simulink model "EL6243_Project_Simulink"  (R2013a)
settings: Solver=ode45  StartTime=0.0  StopTime=60  RelTol=1e-3
libraries: cstblocks x12
settings Model: Creator=pk  LastModifiedBy=meetm_000
settings DataIOCC: SignalLoggingSaveFormat=ModelDataLogs
settings OptimizationCC: InitFltsAndDblsToZero=on
settings DebuggingCC: SaveWithParameterizedLinksMsg=none  SignalResolutionControl=TryResolveAllWithWarning  MultiTaskDSMMsg=warning  MultiTaskCondExecSysMsg=none  StrictBusMsg=None
settings RTWCC: IncludeERTFirstTime=on
settings GRTTargetCC: TargetFcnLib=ansi_tfl_tmw.mat  CombineOutputUpdateFcns=off  GRTInterface=on

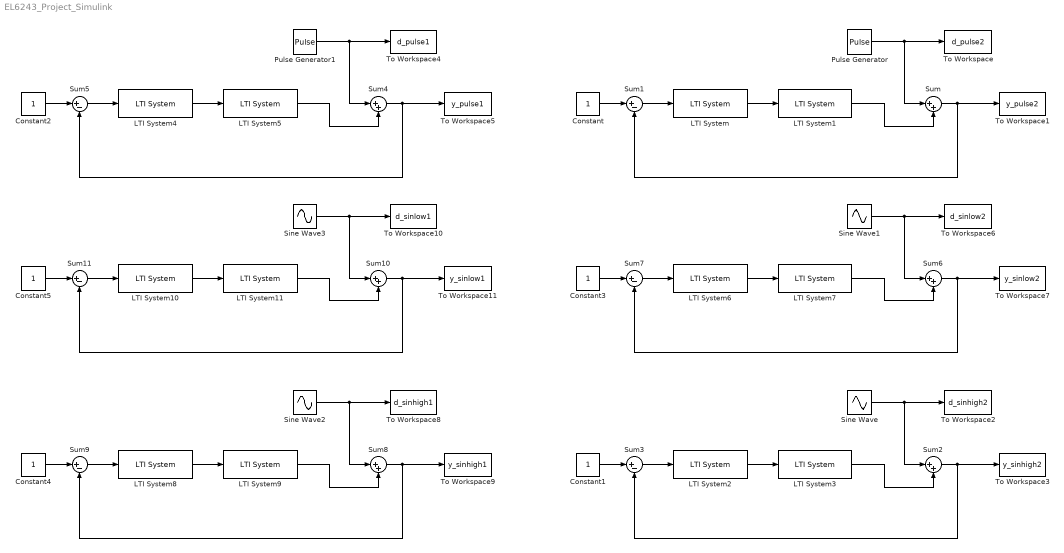
== system EL6243_Project_Simulink ==
  Constant{,1..5} (6 alike) : Constant
  LTI System : cstblocks/LTI System  sys=Gco  IC=[]
  LTI System{1,3,5,7,9,11} (6 alike) : cstblocks/LTI System  sys=Gp  IC=[]
  LTI System10 : cstblocks/LTI System  sys=Gc  IC=[]
  LTI System2 : cstblocks/LTI System  sys=Gco  IC=[]
  LTI System4 : cstblocks/LTI System  sys=Gc  IC=[]
  LTI System6 : cstblocks/LTI System  sys=Gco  IC=[]
  LTI System8 : cstblocks/LTI System  sys=Gc  IC=[]
  Pulse Generator : DiscretePulseGenerator  PulseType=Time based  Period=100  PhaseDelay=40
  Pulse Generator1 : DiscretePulseGenerator  PulseType=Time based  Period=100  PhaseDelay=40
  Sine Wave : Sin  Frequency=10*pi  SampleTime=0
  Sine Wave1 : Sin  Amplitude=0.2  SampleTime=0
  Sine Wave2 : Sin  Frequency=10*pi  SampleTime=0
  Sine Wave3 : Sin  Amplitude=0.2  SampleTime=0
  Sum{,2,4,6,8,10} (6 alike) : Sum  Inputs=|++
  Sum{1,3,5,7,9,11} (6 alike) : Sum  Inputs=|+-
  To Workspace : ToWorkspace  VariableName=d_pulse2  SampleTime=0.01  SaveFormat=Structure With Time
  To Workspace1 : ToWorkspace  VariableName=y_pulse2  SampleTime=0.01  SaveFormat=Structure With Time
  To Workspace10 : ToWorkspace  VariableName=d_sinlow1  SampleTime=0.01  SaveFormat=Structure With Time
  To Workspace11 : ToWorkspace  VariableName=y_sinlow1  SampleTime=0.01  SaveFormat=Structure With Time
  To Workspace2 : ToWorkspace  VariableName=d_sinhigh2  SampleTime=0.01  SaveFormat=Structure With Time
  To Workspace3 : ToWorkspace  VariableName=y_sinhigh2  SampleTime=0.01  SaveFormat=Structure With Time
  To Workspace4 : ToWorkspace  VariableName=d_pulse1  SampleTime=0.01  SaveFormat=Structure With Time
  To Workspace5 : ToWorkspace  VariableName=y_pulse1  SampleTime=0.01  SaveFormat=Structure With Time
  To Workspace6 : ToWorkspace  VariableName=d_sinlow2  SampleTime=0.01  SaveFormat=Structure With Time
  To Workspace7 : ToWorkspace  VariableName=y_sinlow2  SampleTime=0.01  SaveFormat=Structure With Time
  To Workspace8 : ToWorkspace  VariableName=d_sinhigh1  SampleTime=0.01  SaveFormat=Structure With Time
  To Workspace9 : ToWorkspace  VariableName=y_sinhigh1  SampleTime=0.01  SaveFormat=Structure With Time
  wires:
  LTI System/1 -> LTI System1/1
  LTI System1/1 -> Sum/2
  Pulse Generator/1 -> To Workspace/1, Sum/1
  Constant/1 -> Sum1/1
  Sum1/1 -> LTI System/1
  Sum/1 -> To Workspace1/1, Sum1/2
  LTI System2/1 -> LTI System3/1
  LTI System3/1 -> Sum2/2
  Sine Wave/1 -> To Workspace2/1, Sum2/1
  Constant1/1 -> Sum3/1
  Sum3/1 -> LTI System2/1
  Sum2/1 -> To Workspace3/1, Sum3/2
  LTI System6/1 -> LTI System7/1
  LTI System7/1 -> Sum6/2
  Sine Wave1/1 -> To Workspace6/1, Sum6/1
  Constant3/1 -> Sum7/1
  Sum7/1 -> LTI System6/1
  Sum6/1 -> To Workspace7/1, Sum7/2
  LTI System4/1 -> LTI System5/1
  LTI System5/1 -> Sum4/2
  Pulse Generator1/1 -> To Workspace4/1, Sum4/1
  Constant2/1 -> Sum5/1
  Sum5/1 -> LTI System4/1
  Sum4/1 -> To Workspace5/1, Sum5/2
  LTI System8/1 -> LTI System9/1
  LTI System9/1 -> Sum8/2
  Sine Wave2/1 -> To Workspace8/1, Sum8/1
  Constant4/1 -> Sum9/1
  Sum9/1 -> LTI System8/1
  Sum8/1 -> To Workspace9/1, Sum9/2
  LTI System10/1 -> LTI System11/1
  LTI System11/1 -> Sum10/2
  Sine Wave3/1 -> To Workspace10/1, Sum10/1
  Constant5/1 -> Sum11/1
  Sum11/1 -> LTI System10/1
  Sum10/1 -> To Workspace11/1, Sum11/2
